simulink model "fuzzzzzyyyy"  (R2017b)
settings: Solver=FixedStepAuto  StartTime=0.0  StopTime=100  FixedStep=0.01  RelTol=1e-3
values from neighbouring files (symbols this model uses):
  K1 = par(bestchrom,1)    [GA_FUZZY.m]    (also in test_timK.m = par(bestchrom,1)-500; thongsoK_funzzy.m = 5)
  K2 = par(bestchrom,2)    [GA_FUZZY.m]    (also in test_timK.m = par(bestchrom,2)-500; thongsoK_funzzy.m = 2)
  K3 = par(bestchrom,3)    [GA_FUZZY.m]    (also in test_timK.m = par(bestchrom,3)-500; thongsoK_funzzy.m = -7.3)
  K4 = par(bestchrom,4)    [GA_FUZZY.m]    (also in test_timK.m = par(bestchrom,4)-500; thongsoK_funzzy.m = 32)
  K5 = par(bestchrom,5)    [GA_FUZZY.m]    (also in test_timK.m = par(bestchrom,5)-500; thongsoK_funzzy.m = -20)
  q1_d_init = 0.0001    [goc_init.m]
  q2_d_init = 0.02    [goc_init.m]
  q2_init = 0.007    [goc_init.m]
libraries: fuzblock x1
settings Model: Creator=DELL  LastModifiedBy=DELL

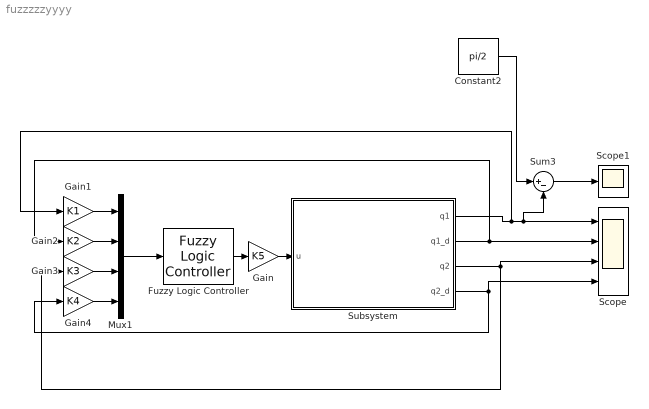
== system fuzzzzzyyyy ==
  Constant2 : Constant  Value=pi/2
  Fuzzy Logic Controller : fuzblock/Fuzzy Logic  Controller  FIS='file_mo_goc_con_lac.fis'  OutputSampleNumber=101  DataType=double  FuzzifiedInputs=off  RuleFiringStrengths=off  RuleOutputs=off  AggregatedOutputs=off  SimulateUsing=Interpreted execution
  Gain : Gain  Gain=K5
  Gain1 : Gain  Gain=K1
  Gain2 : Gain  Gain=K2
  Gain3 : Gain  Gain=K3
  Gain4 : Gain  Gain=K4
  Mux1 : Mux
  Scope : Scope  NumInputPorts=4
  Scope1 : Scope
  Subsystem : Subsystem
  Sum3 : Sum  Inputs=|+-
  wires:
  Subsystem/1(q1) -> Gain1/1, Sum3/2, Scope/1
  Subsystem/2(q1_d) -> Scope/2, Gain2/1
  Subsystem/3(q2) -> Scope/3, Gain3/1
  Subsystem/4(q2_d) -> Scope/4, Gain4/1
  Gain/1 -> Subsystem/1(u)
  Fuzzy Logic Controller/1 -> Gain/1
  Mux1/1 -> Fuzzy Logic Controller/1
  Gain1/1 -> Mux1/1
  Gain2/1 -> Mux1/2
  Gain3/1 -> Mux1/3
  Gain4/1 -> Mux1/4
  Constant2/1 -> Sum3/1
  Sum3/1 -> Scope1/1

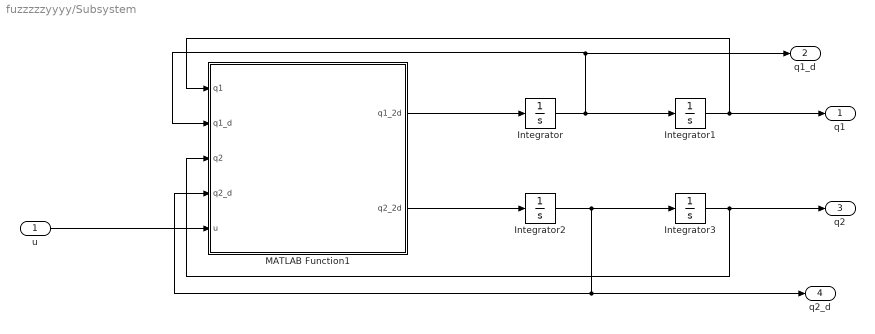
== system fuzzzzzyyyy/Subsystem ==
  u : Inport
  Integrator : Integrator  InitialCondition=q1_d_init
  Integrator1 : Integrator  InitialCondition=pi/2+0.001
  Integrator2 : Integrator  InitialCondition=q2_d_init
  Integrator3 : Integrator  InitialCondition=q2_init
  MATLAB Function1 : MATLAB Function  TreatAsAtomicUnit=on
  q1 : Outport
  q1_d : Outport  Port=2
  q2 : Outport  Port=3
  q2_d : Outport  Port=4
  wires:
  Integrator2/1 -> q2_d/1, MATLAB Function1/4(q2_d), Integrator3/1
  Integrator3/1 -> MATLAB Function1/3(q2), q2/1
  Integrator/1 -> MATLAB Function1/2(q1_d), q1_d/1, Integrator1/1
  u/1 -> MATLAB Function1/5(u)
  MATLAB Function1/2(q2_2d) -> Integrator2/1
  Integrator1/1 -> MATLAB Function1/1(q1), q1/1
  MATLAB Function1/1(q1_2d) -> Integrator/1

== matlab function fuzzzzzyyyy/Subsystem/MATLAB Function1 ==
  data: q1 input; q1_2d output; q1_d input; q2 input; q2_d input; u input; q2_2d output
function [q1_2d,q2_2d] = fcn(q1,q1_d,q2,q2_d,u)
m1=1.068;
m2=0.07;
l1=0.146;
l2=0.253;
lc1=0.055;
lc2=0.149;
I1=0.0189;
I2=0.000409;
Kb=0.0864;
Kt=0.0864;
Rm=3.7;
Cm=0.000415;
Jm=0.000427;
g=9.80665;
K1=Kt/Rm;
K2=((Kt*Kb)/Rm)+Cm;
K3=Jm;
beta1=m1*lc1^2+m2*l1^2+I1;
beta2=m2*lc2^2+I2;
beta3=m2*l1*lc2;
beta4=m1*lc1+m2*l1;
beta5=m2*lc2;
q1_2d=1/(beta1*beta2-beta3^2*(cos(q2))^2+K3*beta2)*(beta2*beta3*sin(q2)*(q1_d+q2_d)^2+beta3^2*cos(q2)*sin(q2)*q1_d^2-beta2*beta4*g*cos(q1)+beta3*beta5*g*cos(q2)*cos(q1+q2)+beta2*K1*u-K2*beta2*q1_d);
%q2_2d=-(2*beta3^2*q1_d^2*sin(2*q2) + beta3^2*q2_d^2*sin(2*q2) - 2*K2*beta2*q1_d + 2*K1*beta2*u + 2*K3*beta5*g*cos(q1 + q2) + 2*beta1*beta5*g*cos(q1 + q2) - beta3*beta4*g*cos(q1 + q2) + 2*beta3^2*q1_d*q2_d*sin(2*q2) - 2*K2*beta3*q1_d*cos(q2) + 2*K1*beta3*u*cos(q2) - 2*beta2*beta4*g*cos(q1) + beta3*beta5*g*cos(q1) - beta3*beta4*g*cos(q1 - q2) + beta3*beta5*g*cos(q1 + 2*q2) + 2*K3*beta3*q1_d^2*sin(q2) + 2*beta1*beta3*q1_d^2*sin(q2) + 2*beta2*beta3*q1_d^2*sin(q2) + 2*beta2*beta3*q2_d^2*sin(q2) + 4*beta2*beta3*q1_d*q2_d*sin(q2))/(2*K3*beta2 + 2*beta1*beta2 - beta3^2*cos(2*q2) - beta3^2);
q2_2d=-(beta5*g*cos(q1 + q2)*(K3 + beta1 + beta3*cos(q2)) - beta4*g*cos(q1)*(beta2 + beta3*cos(q2)) - K2*q1_d*(beta2 + beta3*cos(q2)) + beta3*sin(q2)*(q1_d + q2_d)^2*(beta2 + beta3*cos(q2)) + K3*beta3*q1_d^2*sin(q2) + beta3*q1_d^2*sin(q2)*(beta1 + beta3*cos(q2)))/(- beta3^2*cos(q2)^2 + K3*beta2 + beta1*beta2) - (K1*u*(beta2 + beta3*cos(q2)))/(- beta3^2*cos(q2)^2 + K3*beta2 + beta1*beta2);
